simulink model "Sim4_EndEffector_OA"  (R2021b)
settings: Solver=VariableStepAuto  StartTime=0.0  StopTime=Inf  RelTol=1e-3
PreLoadFcn:
  | %GUI = evalin('base','GUI_handle');
InitFcn:
  | run('settingParams.m')
  | %GUI = evalin('base','GUI_handle');
undefined symbols (not defined in the file or in its folder): dt, Twist
libraries: robotlib x3, instrumentseriallib x3
CloseFcn:
  | %set(findobj(GUI,'Tag','open_sim4'),'Value','Close');
  | %set(findobj(GUI,'Tag','open_sim4'),'Enable','on');
  | %set(findobj(GUI,'Tag','start_sim4'),'Value','Stop');
  | %set(findobj(GUI,'Tag','start_sim4'),'Enable','off');
settings Model: Creator=shdet  LastModifiedBy=Hibik
settings SolverCC: AlgebraicLoopSolver=TrustRegion
settings DataIOCC: ReturnWorkspaceOutputs=off
settings DebuggingCC: PregeneratedLibrarySubsystemCodeDiagnostic=none  SFMachineParentedDataDiag=warning  ArithmeticOperatorsInVariantConditions=warning
settings SFSimCC: SimUseLocalCustomCode=off  CustomCodeUndefinedFunction=UseInterfaceOnly
settings RTWCC: RTWUseLocalCustomCode=off

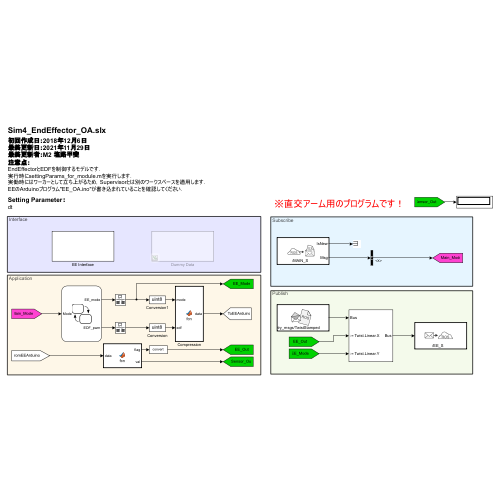
[thumbnail: Simulink's stored preview of the top-level diagram]
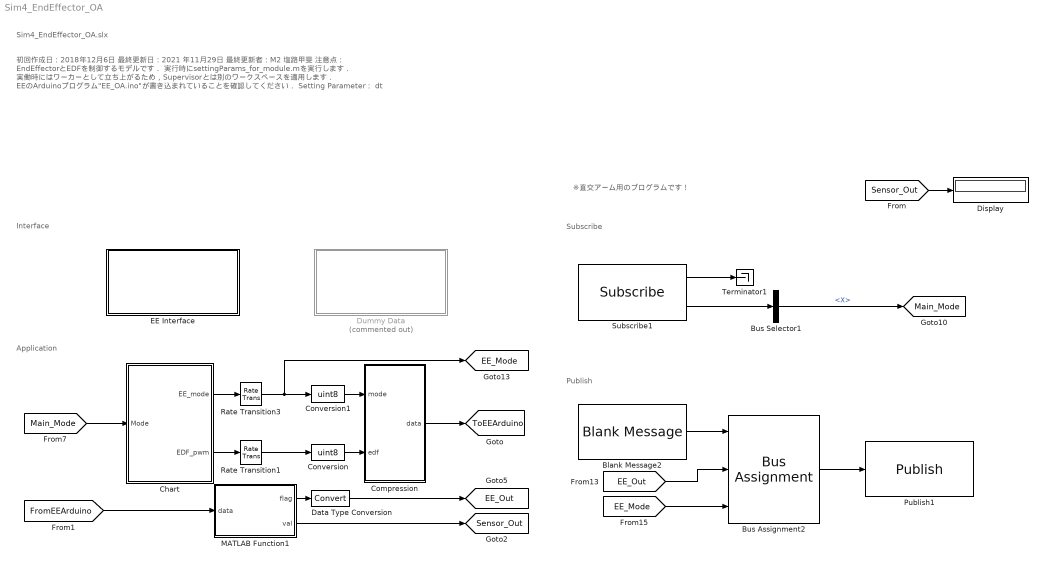
== system Sim4_EndEffector_OA ==
  note: Subscribe
  note: Sim4_EndEffector_OA.slx
  note: ※直交アーム用のプログラムです！
  note: Publish
  note: Application
  note: Interface
  note: 初回作成日：2018年12月6日
      | 最終更新日：2021 年11月29日
      | 最終更新者：M2 塩路甲斐
      | 注意点：
      | EndEffectorとEDFを制御するモデルです．
      | 実行時にsettingParams_for_module.mを実行します．
      | 実働時にはワーカーとして立ち上がるため，Supervisorとは別のワークスペースを適用します．
      | EEのArduinoプログラム"EE_OA.ino"が書き込まれていることを確認してください．
      |
      | Setting Parameter：
      | dt
  Blank Message2 : robotlib/Blank Message  messageClass=Message  entityType=geometry_msgs/TwistStamped  messageType=geometry_msgs/TwistStamped  SampleTime=dt  legacyBusStruct=off
  Bus Assignment2 : BusAssignment  AssignedSignals=Twist.Linear.X,Twist.Linear.Y
  Bus Selector1 : BusSelector  OutputSignals=Twist.Linear.X
  Chart : Stateflow chart  TreatAsAtomicUnit=on
  Compression : MATLAB Function  TreatAsAtomicUnit=on
  Conversion : DataTypeConversion  OutDataTypeStr=uint8
  Conversion1 : DataTypeConversion  OutDataTypeStr=uint8
  Data Type Conversion : DataTypeConversion
  Display : Display
  Dummy Data : Subsystem  Commented=on
  EE Interface : Subsystem
  MATLAB Function1 : MATLAB Function  TreatAsAtomicUnit=on
  Publish1 : robotlib/Publish  topicSource=Specify your own  topic=/EE_S  messageType=geometry_msgs/TwistStamped  legacyBusStruct=off  messageQueueLength=1
  Rate Transition1 : RateTransition  OutPortSampleTime=0.1
  Rate Transition3 : RateTransition  OutPortSampleTime=0.1
  Subscribe1 : robotlib/Subscribe  topicSource=Specify your own  topic=/MAIN_S  messageType=geometry_msgs/TwistStamped  SampleTime=dt  legacyBusStruct=off  messageQueueLength=1
  Terminator1 : Terminator
  tag scope: EE_Mode=global, EE_Out=global, Main_Mode=global, Sensor_Out=global, ToEEArduino=global
  wires:
  [Main_Mode] -> Chart/1(Mode)
  Subscribe1/2 -> Bus Selector1/1
  Conversion/1 -> Compression/2(edf)
  MATLAB Function1/1(flag) -> Data Type Conversion/1
  Subscribe1/1 -> Terminator1/1
  Rate Transition3/1 -> [EE_Mode], Conversion1/1
  Chart/1(EE_mode) -> Rate Transition3/1
  [FromEEArduino] -> MATLAB Function1/1(data)
  Blank Message2/1 -> Bus Assignment2/1
  [EE_Out] -> Bus Assignment2/2
  Chart/2(EDF_pwm) -> Rate Transition1/1
  Bus Assignment2/1 -> Publish1/1
  Bus Selector1/1 -> [Main_Mode]  "<X>"
  MATLAB Function1/2(val) -> [Sensor_Out]
  [EE_Mode] -> Bus Assignment2/3
  Data Type Conversion/1 -> [EE_Out]
  Compression/1(data) -> [ToEEArduino]
  Conversion1/1 -> Compression/1(mode)
  Rate Transition1/1 -> Conversion/1
  [Sensor_Out] -> Display/1

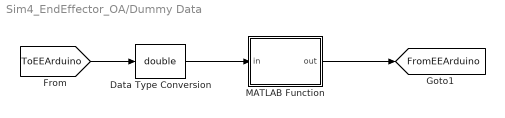
== system Sim4_EndEffector_OA/Dummy Data ==
  Data Type Conversion : DataTypeConversion  OutDataTypeStr=double
  MATLAB Function : MATLAB Function  TreatAsAtomicUnit=on
  tag scope: FromEEArduino=global
  wires:
  MATLAB Function/1(out) -> [FromEEArduino]
  [ToEEArduino] -> Data Type Conversion/1
  Data Type Conversion/1 -> MATLAB Function/1(in)

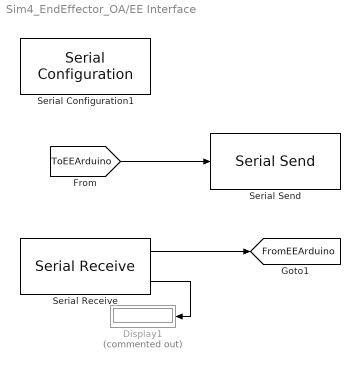
== system Sim4_EndEffector_OA/EE Interface ==
  Display1 : Display  Commented=on
  Serial Configuration1 : instrumentseriallib/Serial Configuration  Priority=-200000  Port=COM6  ComPort=COM6  BaudRate=115200  DataBits=8  Parity=none  StopBits=1  ByteOrder=little-endian  FlowControl=none  Timeout=50  SimulateUsing=Interpreted execution  BlockInModel=on
  Serial Receive : instrumentseriallib/Serial Receive  Priority=1  Port=COM6  ComPort=COM6  DataType=uint8  SaveDataType=uint8  ToggleHeader=off  Header=[]  ToggleTerminator=on  Terminator=<none>  CustomTerminator=[]  ToggleDataSize=on  DataSize=1  EnableBlockingMode=off  ActionDataUnavailable=Output last received value  ActionWhenDataUnavailable=Output last received value  CustomValue=0  SampleTime=0.1  SimulateUsing=Interpreted execution  BlockInModel=on
  Serial Send : instrumentseriallib/Serial Send  Priority=1  Port=COM6  ComPort=COM6  Header=[]  Terminator=<none>  CustomTerminator=[]  EnableBlockingMode=off  SimulateUsing=Interpreted execution  BlockInModel=on
  tag scope: FromEEArduino=global
  wires:
  Serial Receive/1 -> [FromEEArduino]
  Serial Receive/2 -> Display1/1
  [ToEEArduino] -> Serial Send/1

== matlab function Sim4_EndEffector_OA/Dummy Data/MATLAB Function ==
  data: in input; out output
function out = fcn(in)

switch in
    case 0
        data = 0;
    case 1
        data = 5;
    case 2
        data = 6;
    case 3
        data = 7;
    case 4
        data = 4;
    otherwise
        data = 0;
end

out = uint8(bitshift(data,5));

== stateflow chart Sim4_EndEffector_OA/Chart ==
  note: EE_mode0 待機
      | EE_mode1 吸引指令
      | EE_mode2 EE閉じる（吸引）
      | EE_mode3 EE開く（吸引）
      | EE_mode4 閉じたままホールド
  note: Mode42 EE吸引
      | Mode43 光センサ
      |
      | Mode45 上EESW反応
      | Mode61 把持成功
      |
      |
      | Mode47 収穫失敗
      | Mode70 終了モード
  state m03/
    % 切断2_逆転中
    entry:
    EE_mode=3;
    EDF_pwm=17;
  state m0/
    % 待機中
    entry:
    EE_mode=0;
    EDF_pwm=0;
  state m01/
    % 吸引中
    entry:
    EE_mode=1;
    EDF_pwm=19;
  state m04/
    % 把持中
    entry:
    EE_mode=4;
    EDF_pwm=18;
  state m02/
    % 切断1_正転中
    entry:
    EE_mode=2;
    EDF_pwm=20;
  m03 -> m0 : [Mode==47 || Mode==70]
  (default) -> m0
  m02 -> m0 [order 2] : [Mode==47 || Mode==70]
  m04 -> m0 [order 1] : [Mode==47 || Mode==70]
  m01 -> m0 [order 2] : % 失敗
      | [Mode == 47 || Mode == 70]
  m04 -> m03 [order 2] : % 把持成功
      | [Mode == 61]
  m0 -> m01 : % 吸引開始
      | [Mode == 42]
  m01 -> m02 [order 1] : % 光センサ反応
      | [Mode == 43]
  m02 -> m04 [order 1] : % 上SW反応
      | [Mode == 45]
  data: Mode input; EE_mode output; EDF_pwm output

== matlab function Sim4_EndEffector_OA/Compression ==
  data: mode input; edf input; data output
function data = fcn(mode, edf)

if mode < 0
    mode = uint8(0);
elseif mode > 7
    mode = uint8(7);
end

if edf > 25
    edf = uint8(25);
end

pwm = uint8(edf);

data = bitshift(mode,5) + pwm;

== matlab function Sim4_EndEffector_OA/MATLAB Function1 ==
  data: flag output; data input; val output
function [flag,val] = fcn(data)

% 入力(data)を右に5bitシフトして、上位3bitを取り出す
flag = uint8(bitshift(data,-4));

% 入力(data)と31(00011111)のAND演算をして、下位5bitを取り出す
a = double( bitand(data, 15));

val = (a + 41) * 20;
